simulink model "spring_mass_damper_simu_2"  (R2025b)
settings: Solver=ode45  StartTime=0.0  StopTime=2  MaxStep=1e-4  RelTol=1e-3
values from neighbouring files (symbols this model uses):
  A = [ ... (first row only)    [Lab_1.m]
  B = [0; 0; 0; 1/J1; 0; 0]    [Lab_1.m]
  C = [0 0 1 0 0 0]    [Lab_1.m]
undefined symbols (not defined in the file or in its folder): F, K, V
settings Model: Creator=DemoBox  LastModifiedBy=DemoBox

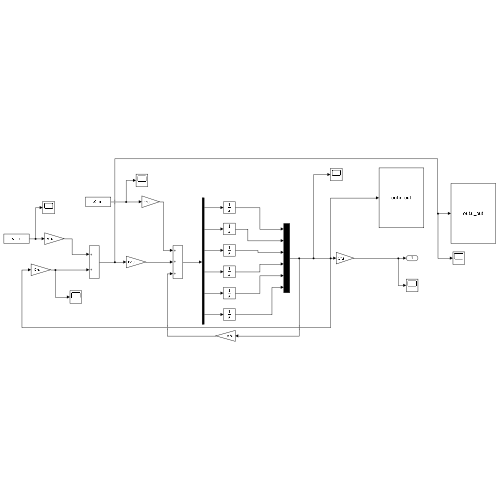
[thumbnail: Simulink's stored preview of the top-level diagram]
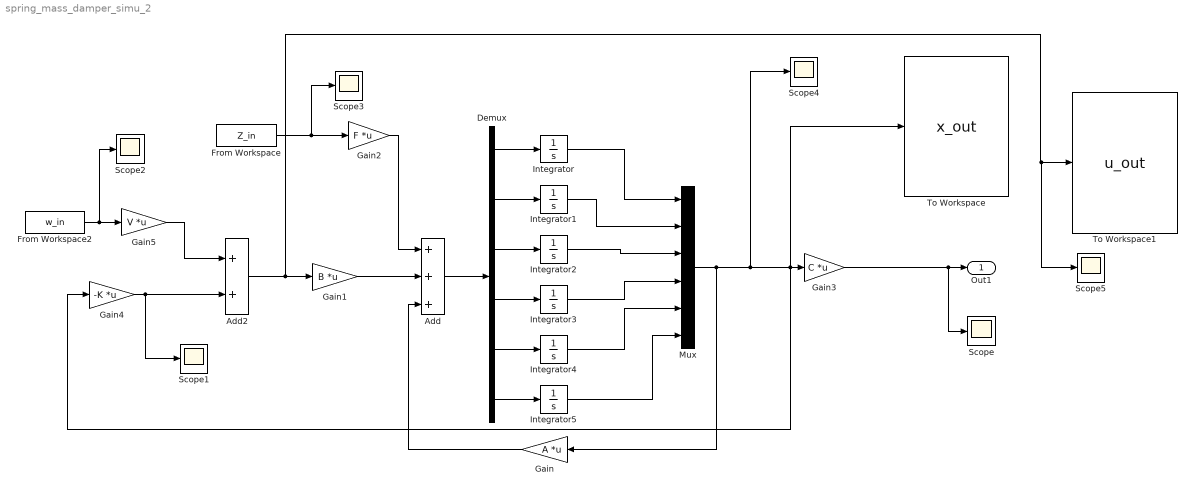
== system spring_mass_damper_simu_2 ==
  Add : Sum  Inputs=+++
  Add2 : Sum
  Demux : Demux  Outputs=6
  From Workspace : FromWorkspace  VariableName=Z_in
  From Workspace2 : FromWorkspace  VariableName=w_in
  Gain : Gain  Gain=A  Multiplication=Matrix(K*u)
  Gain1 : Gain  Gain=B  Multiplication=Matrix(K*u)
  Gain2 : Gain  Gain=F  Multiplication=Matrix(K*u)
  Gain3 : Gain  Gain=C  Multiplication=Matrix(K*u)
  Gain4 : Gain  Gain=-K  Multiplication=Matrix(K*u)
  Gain5 : Gain  Gain=V  Multiplication=Matrix(K*u)
  Integrator{,1..5} (6 alike) : Integrator
  Mux : Mux  Inputs=6
  Scope{,1..5} (6 alike) : Scope
      Scope settings: ActiveDisplayYMinimum=-0.40332105897607384  ActiveDisplayYMaximum=34.149512982524726
      Scope1 settings: ActiveDisplayYMinimum=-8.4680820608434431  ActiveDisplayYMaximum=9.8560235566679513
      Scope2 settings: ActiveDisplayYMinimum=-106.52024630419052  ActiveDisplayYMaximum=58.489977033060882  DataLoggingVariableName=ScopeData2
      Scope3 settings: ActiveDisplayYMinimum=-4.2900357463482344  ActiveDisplayYMaximum=3.8362712639379692  DataLoggingVariableName=ScopeData3
      Scope4 settings: ActiveDisplayYMinimum=-4.2900357463482344  ActiveDisplayYMaximum=3.8362712639379692  DataLoggingVariableName=ScopeData4
      Scope5 settings: ActiveDisplayYMinimum=-4.2900357463482344  ActiveDisplayYMaximum=3.8362712639379692  DataLoggingVariableName=ScopeData5
  To Workspace : ToWorkspace  VariableName=x_out  SaveFormat=Structure With Time  SampleTime=-1
  To Workspace1 : ToWorkspace  VariableName=u_out  SaveFormat=Structure With Time  SampleTime=-1
  Out1 : Outport
  wires:
  Integrator/1 -> Mux/1
  Integrator1/1 -> Mux/2
  Integrator2/1 -> Mux/3
  Integrator3/1 -> Mux/4
  Integrator4/1 -> Mux/5
  Integrator5/1 -> Mux/6
  Mux/1 -> Scope4/1, Gain4/1, To Workspace/1, Gain3/1, Gain/1
  Gain2/1 -> Add/1
  Gain1/1 -> Add/2
  Gain/1 -> Add/3
  Add/1 -> Demux/1
  Demux/1 -> Integrator/1
  Demux/2 -> Integrator1/1
  Demux/3 -> Integrator2/1
  Demux/4 -> Integrator3/1
  Demux/5 -> Integrator4/1
  Demux/6 -> Integrator5/1
  Gain3/1 -> Scope/1, Out1/1
  From Workspace/1 -> Scope3/1, Gain2/1
  From Workspace2/1 -> Scope2/1, Gain5/1
  Gain4/1 -> Scope1/1, Add2/2
  Add2/1 -> Scope5/1, To Workspace1/1, Gain1/1
  Gain5/1 -> Add2/1
